simulink model "linear_sim"  (R2025a)
settings: Solver=VariableStepAuto  StartTime=0.0  StopTime=10.0  RelTol=1e-3
settings Model: Creator=henri  LastModifiedBy=guilherme-lazzarini

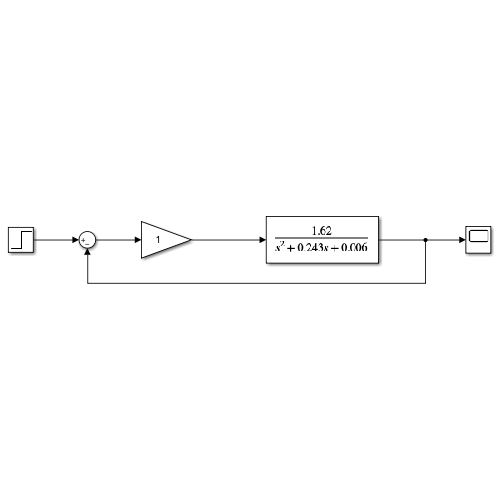
[thumbnail: Simulink's stored preview of the top-level diagram]
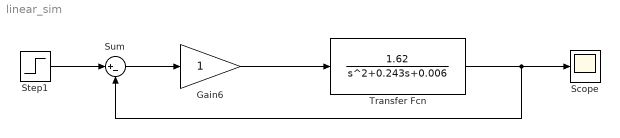
== system linear_sim ==
  Gain6 : Gain
  Scope : Scope
      settings: ActiveDisplayYMinimum=-4.4434687533166048  ActiveDisplayYMaximum=39.991218779849454
  Step1 : Step  Time=0.8  SampleTime=0
  Sum : Sum  Inputs=|+-
  Transfer Fcn : TransferFcn  Numerator=[1.62]  Denominator=[1 0.243 0.006]
  wires:
  Gain6/1 -> Transfer Fcn/1
  Transfer Fcn/1 -> Sum/2, Scope/1
  Step1/1 -> Sum/1
  Sum/1 -> Gain6/1
